simulink model "wind_and_turb_comparison"  (Simulink 7.6)
settings: Solver=FixedStepDiscrete  SolverMode=SingleTasking  StartTime=0.0  StopTime=49.99  FixedStep=0.01  RelTol=1e-3
values from neighbouring files (symbols this model uses):
  r = - obj.PENALTY    [TaskCompareWindWithSimulink.m]    (also in TaskCompareWindWithSimulinkW2D0.m; TaskCompareWindWithSimulinkW2D30.m; TaskCompareWindWithSimulinkW2D90.m)
undefined symbols (not defined in the file or in its folder): F, MIL, Moderate
libraries: aerolibwind2 x2, aerolibtransform2 x1
settings Model: Creator=rdenardi  LastModifiedBy=rdenardi
settings DataIOCC: ExternalInput=simin  LimitDataPoints=off  LoadExternalInput=on  SignalLogging=off  DSMLogging=off

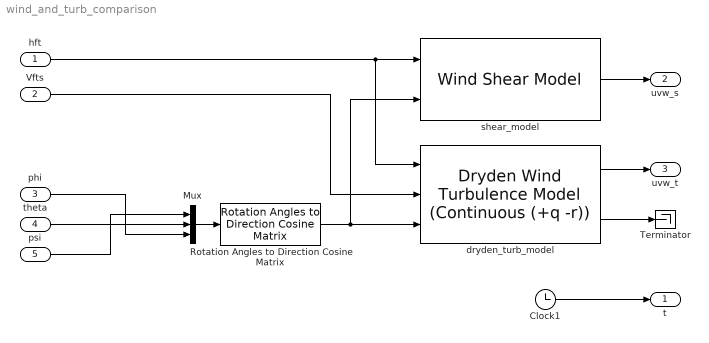
== system wind_and_turb_comparison ==
  hft : Inport
  Vfts : Inport  Port=2
  phi : Inport  Port=3
  theta : Inport  Port=4
  psi : Inport  Port=5
  Clock1 : Clock
      settings: Decimation=10
  Mux : Mux  Inputs=3
  Rotation Angles to Direction Cosine Matrix : aerolibtransform2/Rotation Angles to Direction Cosine Matrix  SystemSampleTime=-1  rotationOrder=ZYX
  Terminator : Terminator
  dryden_turb_model : aerolibwind2/Dryden Wind Turbulence Model  (Continuous (+q -r))  SystemSampleTime=-1  units=English (Velocity in ft/s)  spec=MIL-F-8785C  model=Discrete Dryden (+q +r)  W20=20  Wdeg=30  TurbProb=10^-3 - Moderate  L_high=1000  Wingspan=0.5  ts=0.01  Seed=[23341 23342 23343 23344]  T_on=on
  shear_model : aerolibwind2/Wind Shear Model  SystemSampleTime=-1  units=English (Velocity in ft/s)  phase=Category C - Terminal Flight Phase  W_20=10  Wdeg=0
  t : Outport
  uvw_s : Outport  Port=2
  uvw_t : Outport  Port=3
  wires:
  dryden_turb_model/2 -> Terminator/1
  Mux/1 -> Rotation Angles to Direction Cosine Matrix/1
  dryden_turb_model/1 -> uvw_t/1
  shear_model/1 -> uvw_s/1
  hft/1 -> shear_model/1, dryden_turb_model/1
  Vfts/1 -> dryden_turb_model/2
  phi/1 -> Mux/3
  theta/1 -> Mux/2
  psi/1 -> Mux/1
  Clock1/1 -> t/1
  Rotation Angles to Direction Cosine Matrix/1 -> dryden_turb_model/3, shear_model/2
